simulink model "PV_model"  (R2020b)
settings: Solver=FixedStepAuto  StartTime=0.0  StopTime=24  FixedStep=1  RelTol=1e-3
values from neighbouring files (symbols this model uses):
  beta_pv = 0.0045    [Parameters.m]
  eta_pv = 0.15    [Parameters.m]
  Npv = 6    [Parameters.m]
  T_NOCT = 45    [Parameters.m]
  T_ref = 25    [Parameters.m]
settings Model: Creator=enzlp  LastModifiedBy=enzlp
settings DataIOCC: ReturnWorkspaceOutputs=off
settings DebuggingCC: ArithmeticOperatorsInVariantConditions=warning
settings SFSimCC: CustomCodeUndefinedFunction=UseInterfaceOnly

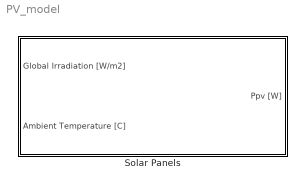
== system PV_model ==
  Solar Panels : Subsystem

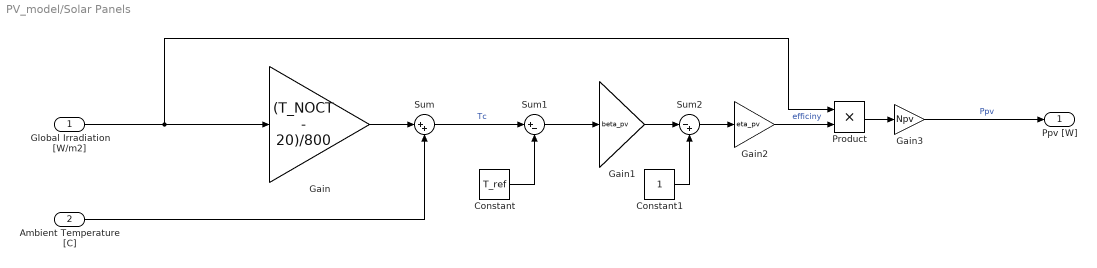
== system PV_model/Solar Panels ==
  Global Irradiation [W/m2] : Inport
  Ambient Temperature [C] : Inport  Port=2
  Constant : Constant  Value=T_ref
  Constant1 : Constant
  Gain : Gain  Gain=(T_NOCT - 20)/800
  Gain1 : Gain  Gain=beta_pv
  Gain2 : Gain  Gain=eta_pv
  Gain3 : Gain  Gain=Npv
  Product : Product
  Sum : Sum  Inputs=|++
  Sum1 : Sum  Inputs=|+-
  Sum2 : Sum  Inputs=|-+
  Ppv [W] : Outport  VectorParamsAs1DForOutWhenUnconnected=off
  wires:
  Gain3/1 -> Ppv [W]/1  "Ppv"
  Sum1/1 -> Gain1/1
  Gain/1 -> Sum/1
  Constant1/1 -> Sum2/2
  Sum/1 -> Sum1/1  "Tc"
  Sum2/1 -> Gain2/1
  Constant/1 -> Sum1/2
  Gain2/1 -> Product/2  "efficiny"
  Gain1/1 -> Sum2/1
  Global Irradiation [W/m2]/1 -> Product/1, Gain/1
  Product/1 -> Gain3/1
  Ambient Temperature [C]/1 -> Sum/2
